simulink model "classifier"  (R2012b)
settings: Solver=ode45  SolverMode=SingleTasking  StartTime=0.0  StopTime=29999  RelTol=1e-3
libraries: xbsIndex_r4 x57
settings Model: Creator=skhay  LastModifiedBy=maolin

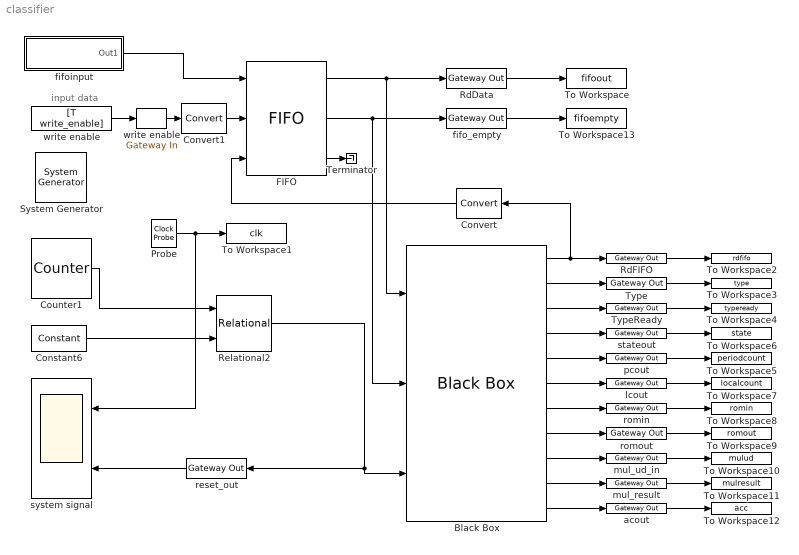
== system classifier ==
  note: input data
  " write enable" : FromWorkspace  VariableName=[T write_enable]  SampleTime=0
  " System Generator" : xbsIndex_r4/ System Generator  Tag=genX  xilinxfamily=virtex6  part=xc6vsx475t  speed=-1  package=ff1759  synthesis_tool=XST  clock_wrapper=Clock Enables  directory=./celldet_ppp_sysgen  proj_type=Project Navigator  Synth_file=XST Defaults  Impl_file=ISE Defaults  testbench=off  simulink_period=1  sysclk_period=5  dcm_input_clock_period=100  incr_netlist=off  trim_vbits=Everywhere in SubSystem  dbl_ovrd=According to Block Masks  core_generation=According to Block Masks  run_coregen=off  deprecated_control=off  eval_field=0  block_type=sysgen
      settings: block_version=11.4
  Black Box : xbsIndex_r4/Black Box  init_code=svm_config  sim_method=ISE Simulator  verbose=off  block_type=blackbox2
  Constant6 : xbsIndex_r4/Constant  const=2  gui_display_data_type=Fixed-point  arith_type=Unsigned  n_bits=8  bin_pt=0  preci_type=Single  exp_width=8  frac_width=24  explicit_period=off  period=1  equ=P=C  opselect=C  inp2=PCIN>>17  opr=+  inp1=P  carry=CIN  dbl_ovrd=off  block_type=constant
  Convert : xbsIndex_r4/Convert  gui_display_data_type=Boolean  arith_type=Boolean  n_bits=16  bin_pt=14  float_type=Single  exp_bits=8  fraction_bits=24  quantization=Truncate  overflow=Wrap  en=off  latency=0  dbl_ovrd=off  pipeline=off  block_type=convert
  Convert1 : xbsIndex_r4/Convert  gui_display_data_type=Boolean  arith_type=Boolean  n_bits=16  bin_pt=14  float_type=Single  exp_bits=8  fraction_bits=24  quantization=Truncate  overflow=Wrap  en=off  latency=0  dbl_ovrd=off  pipeline=off  block_type=convert
  Counter1 : xbsIndex_r4/Counter  cnt_type=Free Running  cnt_to=255  operation=Up  start_count=0  cnt_by_val=1  arith_type=Unsigned  n_bits=16  bin_pt=0  load_pin=off  rst=off  en=off  explicit_period=on  period=1  dbl_ovrd=off  use_behavioral_HDL=off  implementation=Fabric  block_type=counter
  FIFO : xbsIndex_r4/FIFO  mem_type=Block RAM  performance_options=Standard_FIFO  infoedit1=Available only for V4, V5, V6, V7, K7, A7 and Zynq devices.  embedded_registers=off  depth=1K  percent_nbits=1  rst=off  en=off  use_dcount=off  use_percent_full_port=off  use_almost_empty=off  almost_empty_thresh=2  use_almost_full=off  almost_full_thresh=14  dbl_ovrd=off  explicit_period=off  block_type=fifo
  Probe : xbsIndex_r4/Clock Probe  block_type=clkprobe
      settings: infoedit="Clock probe.  Produces an output of type double that mirrors the hardware system clock.<br><br>Hardware notes:  This block is ignored when hardware is generated."
  RdData : xbsIndex_r4/Gateway Out  inherit_from_input=on  hdl_port=off  timing_constraint=None  locs_specified=off  LOCs={}  UseAsDAC=off  DACChannel='1'  block_type=gatewayout
  RdFIFO : xbsIndex_r4/Gateway Out  inherit_from_input=on  hdl_port=off  timing_constraint=None  locs_specified=off  LOCs={}  UseAsDAC=off  DACChannel='1'  block_type=gatewayout
  Relational2 : xbsIndex_r4/Relational  mode=a>=b  en=off  latency=0  dbl_ovrd=off  block_type=relational
  Terminator : Terminator
  To Workspace : ToWorkspace  VariableName=fifoout  SampleTime=-1  SaveFormat=Timeseries
  To Workspace1 : ToWorkspace  VariableName=clk  SampleTime=-1  SaveFormat=Timeseries
  To Workspace10 : ToWorkspace  VariableName=mulud  SampleTime=-1  SaveFormat=Timeseries
  To Workspace11 : ToWorkspace  VariableName=mulresult  SampleTime=-1  SaveFormat=Timeseries
  To Workspace12 : ToWorkspace  VariableName=acc  SampleTime=-1  SaveFormat=Timeseries
  To Workspace13 : ToWorkspace  VariableName=fifoempty  SampleTime=-1  SaveFormat=Timeseries
  To Workspace2 : ToWorkspace  VariableName=rdfifo  SampleTime=-1  SaveFormat=Timeseries
  To Workspace3 : ToWorkspace  VariableName=type  SampleTime=-1  SaveFormat=Timeseries
  To Workspace4 : ToWorkspace  VariableName=typeready  SampleTime=-1  SaveFormat=Timeseries
  To Workspace5 : ToWorkspace  VariableName=periodcount  SampleTime=-1  SaveFormat=Timeseries
  To Workspace6 : ToWorkspace  VariableName=state  SampleTime=-1  SaveFormat=Timeseries
  To Workspace7 : ToWorkspace  VariableName=localcount  SampleTime=-1  SaveFormat=Timeseries
  To Workspace8 : ToWorkspace  VariableName=romin  SampleTime=-1  SaveFormat=Timeseries
  To Workspace9 : ToWorkspace  VariableName=romout  SampleTime=-1  SaveFormat=Timeseries
  Type : xbsIndex_r4/Gateway Out  inherit_from_input=on  hdl_port=off  timing_constraint=None  locs_specified=off  LOCs={}  UseAsDAC=off  DACChannel='1'  block_type=gatewayout
  TypeReady : xbsIndex_r4/Gateway Out  inherit_from_input=on  hdl_port=off  timing_constraint=None  locs_specified=off  LOCs={}  UseAsDAC=off  DACChannel='1'  block_type=gatewayout
  acout : xbsIndex_r4/Gateway Out  inherit_from_input=on  hdl_port=off  timing_constraint=None  locs_specified=off  LOCs={}  UseAsDAC=off  DACChannel='1'  block_type=gatewayout
  fifo_empty : xbsIndex_r4/Gateway Out  inherit_from_input=on  hdl_port=off  timing_constraint=None  locs_specified=off  LOCs={}  UseAsDAC=off  DACChannel='1'  block_type=gatewayout
  fifoinput : Subsystem
  lcout : xbsIndex_r4/Gateway Out  inherit_from_input=on  hdl_port=off  timing_constraint=None  locs_specified=off  LOCs={}  UseAsDAC=off  DACChannel='1'  block_type=gatewayout
  mul_result : xbsIndex_r4/Gateway Out  inherit_from_input=on  hdl_port=off  timing_constraint=None  locs_specified=off  LOCs={}  UseAsDAC=off  DACChannel='1'  block_type=gatewayout
  mul_ud_in : xbsIndex_r4/Gateway Out  inherit_from_input=on  hdl_port=off  timing_constraint=None  locs_specified=off  LOCs={}  UseAsDAC=off  DACChannel='1'  block_type=gatewayout
  pcout : xbsIndex_r4/Gateway Out  inherit_from_input=on  hdl_port=off  timing_constraint=None  locs_specified=off  LOCs={}  UseAsDAC=off  DACChannel='1'  block_type=gatewayout
  reset_out : xbsIndex_r4/Gateway Out  inherit_from_input=on  hdl_port=off  timing_constraint=None  locs_specified=off  LOCs={}  UseAsDAC=off  DACChannel='1'  block_type=gatewayout
  romin : xbsIndex_r4/Gateway Out  inherit_from_input=on  hdl_port=off  timing_constraint=None  locs_specified=off  LOCs={}  UseAsDAC=off  DACChannel='1'  block_type=gatewayout
  romout : xbsIndex_r4/Gateway Out  inherit_from_input=on  hdl_port=off  timing_constraint=None  locs_specified=off  LOCs={}  UseAsDAC=off  DACChannel='1'  block_type=gatewayout
  stateout : xbsIndex_r4/Gateway Out  inherit_from_input=on  hdl_port=off  timing_constraint=None  locs_specified=off  LOCs={}  UseAsDAC=off  DACChannel='1'  block_type=gatewayout
  system signal : Scope  NumInputPorts=2
      settings: ShowLegends=on  YMin=-5~-5  YMax=5~5
  write enable : xbsIndex_r4/Gateway In  gui_display_data_type=Fixed-point  arith_type=Unsigned  n_bits=1  bin_pt=0  preci_type=Single  exp_width=8  frac_width=24  quantization="Round  (unbiased: +/- Inf)"  overflow=Saturate  period=1  dbl_ovrd=off  timing_constraint=None  locs_specified=off  LOCs={}  UseAsADC=off  ADCChannel='1'  inherit_from_input=off  hdl_port=on  block_type=gatewayin
  wires:
  FIFO/1 -> Black Box/1, RdData/1
  FIFO/3 -> Terminator/1
  fifoinput/1(Out1) -> FIFO/1
  RdData/1 -> To Workspace/1
  FIFO/2 -> Black Box/2, fifo_empty/1
  Counter1/1 -> Relational2/1
  Constant6/1 -> Relational2/2
  Black Box/2 -> Type/1
  Black Box/3 -> TypeReady/1
  Convert/1 -> FIFO/3
  Probe/1 -> To Workspace1/1, system signal/1
  reset_out/1 -> system signal/2
  Black Box/1 -> Convert/1, RdFIFO/1
  Black Box/4 -> stateout/1
  Black Box/5 -> pcout/1
  Black Box/6 -> lcout/1
  Black Box/11 -> acout/1
  TypeReady/1 -> To Workspace4/1
  Type/1 -> To Workspace3/1
  RdFIFO/1 -> To Workspace2/1
  Relational2/1 -> Black Box/3, reset_out/1
  stateout/1 -> To Workspace6/1
  pcout/1 -> To Workspace5/1
  lcout/1 -> To Workspace7/1
  acout/1 -> To Workspace12/1
  mul_result/1 -> To Workspace11/1
  mul_ud_in/1 -> To Workspace10/1
  romout/1 -> To Workspace9/1
  romin/1 -> To Workspace8/1
  Black Box/7 -> romin/1
  Black Box/8 -> romout/1
  Black Box/9 -> mul_ud_in/1
  Black Box/10 -> mul_result/1
  " write enable"/1 -> write enable/1
  Convert1/1 -> FIFO/2
  write enable/1 -> Convert1/1
  fifo_empty/1 -> To Workspace13/1

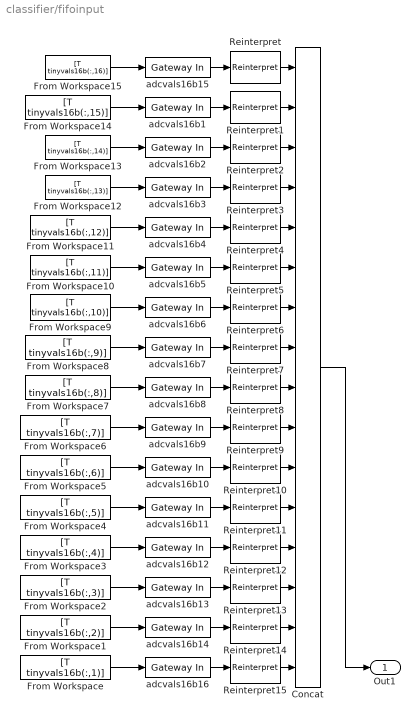
== system classifier/fifoinput ==
  Concat : xbsIndex_r4/Concat  num_inputs=16  dbl_ovrd=off  block_type=concat
  From Workspace : FromWorkspace  VariableName=[T tinyvals16b(:,1)]  SampleTime=1
  From Workspace1 : FromWorkspace  VariableName=[T tinyvals16b(:,2)]  SampleTime=1
  From Workspace10 : FromWorkspace  VariableName=[T tinyvals16b(:,11)]  SampleTime=1
  From Workspace11 : FromWorkspace  VariableName=[T tinyvals16b(:,12)]  SampleTime=1
  From Workspace12 : FromWorkspace  VariableName=[T tinyvals16b(:,13)]  SampleTime=1
  From Workspace13 : FromWorkspace  VariableName=[T tinyvals16b(:,14)]  SampleTime=1
  From Workspace14 : FromWorkspace  VariableName=[T tinyvals16b(:,15)]  SampleTime=1
  From Workspace15 : FromWorkspace  VariableName=[T tinyvals16b(:,16)]  SampleTime=1
  From Workspace2 : FromWorkspace  VariableName=[T tinyvals16b(:,3)]  SampleTime=1
  From Workspace3 : FromWorkspace  VariableName=[T tinyvals16b(:,4)]  SampleTime=1
  From Workspace4 : FromWorkspace  VariableName=[T tinyvals16b(:,5)]  SampleTime=1
  From Workspace5 : FromWorkspace  VariableName=[T tinyvals16b(:,6)]  SampleTime=1
  From Workspace6 : FromWorkspace  VariableName=[T tinyvals16b(:,7)]  SampleTime=1
  From Workspace7 : FromWorkspace  VariableName=[T tinyvals16b(:,8)]  SampleTime=1
  From Workspace8 : FromWorkspace  VariableName=[T tinyvals16b(:,9)]  SampleTime=1
  From Workspace9 : FromWorkspace  VariableName=[T tinyvals16b(:,10)]  SampleTime=1
  Reinterpret{,1..15} (16 alike) : xbsIndex_r4/Reinterpret  force_arith_type=on  arith_type=Unsigned  force_bin_pt=on  bin_pt=0  block_type=reinterpret
  adcvals16b{1..16} (16 alike) : xbsIndex_r4/Gateway In  gui_display_data_type=Fixed-point  arith_type="Signed  (2's comp)"  n_bits=8  bin_pt=0  preci_type=Single  exp_width=8  frac_width=24  quantization="Round  (unbiased: +/- Inf)"  overflow=Saturate  period=1  dbl_ovrd=off  timing_constraint=None  locs_specified=off  LOCs={}  UseAsADC=off  ADCChannel='1'  inherit_from_input=off  hdl_port=on  block_type=gatewayin
  Out1 : Outport
  wires:
  Concat/1 -> Out1/1
  From Workspace15/1 -> adcvals16b15/1
  From Workspace14/1 -> adcvals16b1/1
  From Workspace13/1 -> adcvals16b2/1
  From Workspace12/1 -> adcvals16b3/1
  From Workspace11/1 -> adcvals16b4/1
  From Workspace10/1 -> adcvals16b5/1
  From Workspace9/1 -> adcvals16b6/1
  From Workspace8/1 -> adcvals16b7/1
  From Workspace7/1 -> adcvals16b8/1
  From Workspace6/1 -> adcvals16b9/1
  From Workspace5/1 -> adcvals16b10/1
  From Workspace4/1 -> adcvals16b11/1
  From Workspace3/1 -> adcvals16b12/1
  From Workspace2/1 -> adcvals16b13/1
  From Workspace1/1 -> adcvals16b14/1
  From Workspace/1 -> adcvals16b16/1
  adcvals16b15/1 -> Reinterpret/1
  Reinterpret/1 -> Concat/1
  adcvals16b1/1 -> Reinterpret1/1
  Reinterpret1/1 -> Concat/2
  adcvals16b2/1 -> Reinterpret2/1
  Reinterpret2/1 -> Concat/3
  adcvals16b3/1 -> Reinterpret3/1
  Reinterpret3/1 -> Concat/4
  adcvals16b4/1 -> Reinterpret4/1
  Reinterpret4/1 -> Concat/5
  adcvals16b5/1 -> Reinterpret5/1
  Reinterpret5/1 -> Concat/6
  adcvals16b6/1 -> Reinterpret6/1
  Reinterpret6/1 -> Concat/7
  adcvals16b7/1 -> Reinterpret7/1
  Reinterpret7/1 -> Concat/8
  adcvals16b8/1 -> Reinterpret8/1
  Reinterpret8/1 -> Concat/9
  adcvals16b9/1 -> Reinterpret9/1
  Reinterpret9/1 -> Concat/10
  adcvals16b10/1 -> Reinterpret10/1
  Reinterpret10/1 -> Concat/11
  adcvals16b11/1 -> Reinterpret11/1
  Reinterpret11/1 -> Concat/12
  adcvals16b12/1 -> Reinterpret12/1
  Reinterpret12/1 -> Concat/13
  adcvals16b13/1 -> Reinterpret13/1
  Reinterpret13/1 -> Concat/14
  adcvals16b14/1 -> Reinterpret14/1
  Reinterpret14/1 -> Concat/15
  adcvals16b16/1 -> Reinterpret15/1
  Reinterpret15/1 -> Concat/16
